simulink model "scaler_16bits_v2"  (R2021a)
settings: Solver=VariableStepAuto  StartTime=0.0  StopTime=10.0  RelTol=1e-3
libraries: xbsIndex_r4 x70
settings Model: Creator=11037  LastModifiedBy=11037

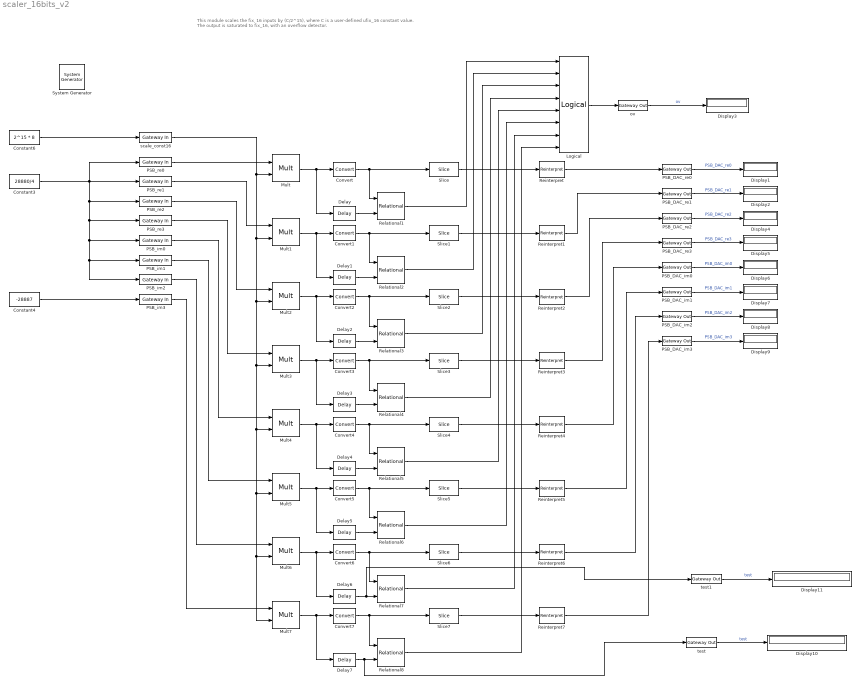
== system scaler_16bits_v2 ==
  note: This module scales the fix_16 inputs by (C/2^15),
      | where C is a user-defined ufix_16 constant value.
      | The output is saturated to fix_16, with an overflow detector.
  " System Generator" : xbsIndex_r4/ System Generator  Tag=genX  xilinxfamily=zynquplusRFSOC  part=xczu28dr  speed=-2-e  package=ffvg1517  synthesis_tool=Vivado  clock_wrapper=Clock Enables  directory=C:/scaler_16bits_v2_NL  proj_type=Vivado  Synth_file=Vivado Synthesis Defaults  Impl_file=Vivado Implementation Defaults  testbench=off  simulink_period=1  sysclk_period=10  dcm_input_clock_period=10  incr_netlist=off  trim_vbits=Everywhere in SubSystem  dbl_ovrd=According to Block Masks  core_generation=According to Block Masks  run_coregen=off  deprecated_control=off  eval_field=0  block_type=sysgen
  Constant3 : Constant  Value=28880/4  SampleTime=1
  Constant4 : Constant  Value=-28887  SampleTime=1
  Constant6 : Constant  Value=2^15 * 8  SampleTime=1
  Convert{,1..7} (8 alike) : xbsIndex_r4/Convert  gui_display_data_type=Fixed-point  arith_type="Signed  (2's comp)"  n_bits=16+15  bin_pt=0  float_type=Single  exp_bits=8  fraction_bits=24  quantization=Truncate  overflow=Saturate  en=off  latency=1  pipeline=off  dbl_ovrd=off  block_type=convert
  Delay{,1..7} (8 alike) : xbsIndex_r4/Delay  rst=off  infoeditControl=Selection of Reset will increase slice count due to use of real FFs and instead of SRLs  en=off  latency=1  reg_retiming=off  dbl_ovrd=off  block_type=delay
  Display{1..11} (11 alike) : Display
      Display1 settings: Format=decimal (Stored Integer)
      Display10 settings: Format=decimal (Stored Integer)
      Display11 settings: Format=decimal (Stored Integer)
      Display2 settings: Format=decimal (Stored Integer)
      Display3 settings: Format=binary (Stored Integer)
      Display4 settings: Format=decimal (Stored Integer)
      Display5 settings: Format=decimal (Stored Integer)
      Display6 settings: Format=decimal (Stored Integer)
      Display7 settings: Format=decimal (Stored Integer)
      Display8 settings: Format=decimal (Stored Integer)
      Display9 settings: Format=decimal (Stored Integer)
  Logical : xbsIndex_r4/Logical  logical_function=OR  inputs=8  en=off  latency=1  precision=User Defined  arith_type=Boolean  n_bits=1  bin_pt=0  align_bp=on  dbl_ovrd=off  block_type=logical
  Mult{,1..7} (8 alike) : xbsIndex_r4/Mult  precision=User Defined  arith_type="Signed  (2's comp)"  n_bits=48  bin_pt=0  quantization=Truncate  overflow=Flag as error  en=off  latency=3  use_behavioral_HDL=off  opt=Speed  use_embedded=on  optimum_pipeline=off  pipeline=on  dbl_ovrd=off  use_rpm=on  placement_style=Triangular  block_type=mult
  PSB_DAC_im{0..3} (4 alike) : xbsIndex_r4/Gateway Out  inherit_from_input=on  hdl_port=on  rows=1  columns=1  UseAsDAC=off  DACChannel='1'  interface=None  automatic_assignment=on  address_offset=hex2dec('00')  intf_name=''  intf_description=''  timing_constraint=None  locs_specified=off  LOCs={}  io_standard={}  block_type=gatewayout
  PSB_DAC_re{0..3} (4 alike) : xbsIndex_r4/Gateway Out  inherit_from_input=on  hdl_port=on  rows=1  columns=1  UseAsDAC=off  DACChannel='1'  interface=None  automatic_assignment=on  address_offset=hex2dec('00')  intf_name=''  intf_description=''  timing_constraint=None  locs_specified=off  LOCs={}  io_standard={}  block_type=gatewayout
  PSB_im{0..3} (4 alike) : xbsIndex_r4/Gateway In  gui_display_data_type=Fixed-point  arith_type="Signed  (2's comp)"  n_bits=16  bin_pt=0  preci_type=Single  exp_width=8  frac_width=24  rows=1  columns=1  quantization=Truncate  overflow=Saturate  period=1  UseAsADC=off  ADCChannel='1'  interface=None  automatic_assignment=on  address_offset=hex2dec('00')  intf_name=''  intf_description=''  default_value=0  timing_constraint=None  locs_specified=off  LOCs={}  io_standard={}  inherit_from_input=off  hdl_port=on  dbl_ovrd=off  block_type=gatewayin
  PSB_re{0..3} (4 alike) : xbsIndex_r4/Gateway In  gui_display_data_type=Fixed-point  arith_type="Signed  (2's comp)"  n_bits=16  bin_pt=0  preci_type=Single  exp_width=8  frac_width=24  rows=1  columns=1  quantization=Truncate  overflow=Saturate  period=1  UseAsADC=off  ADCChannel='1'  interface=None  automatic_assignment=on  address_offset=hex2dec('00')  intf_name=''  intf_description=''  default_value=0  timing_constraint=None  locs_specified=off  LOCs={}  io_standard={}  inherit_from_input=off  hdl_port=on  dbl_ovrd=off  block_type=gatewayin
  Reinterpret{,1..7} (8 alike) : xbsIndex_r4/Reinterpret  force_arith_type=on  arith_type="Signed  (2's comp)"  force_bin_pt=off  bin_pt=0  block_type=reinterpret
  Relational{1..8} (8 alike) : xbsIndex_r4/Relational  mode=a!=b  op_type=Bool  en=off  latency=1  dbl_ovrd=off  block_type=relational
  Slice{,1..7} (8 alike) : xbsIndex_r4/Slice  nbits=16  boolean_output=off  mode=Upper Bit Location + Width  bit1=0  base1=MSB of Input  bit0=0  base0=LSB of Input  dbl_ovrd=off  block_type=slice
  ov : xbsIndex_r4/Gateway Out  inherit_from_input=on  hdl_port=on  rows=1  columns=1  UseAsDAC=off  DACChannel='1'  interface=None  automatic_assignment=on  address_offset=hex2dec('00')  intf_name=''  intf_description=''  timing_constraint=None  locs_specified=off  LOCs={}  io_standard={}  block_type=gatewayout
  scale_const16 : xbsIndex_r4/Gateway In  gui_display_data_type=Fixed-point  arith_type=Unsigned  n_bits=32  bin_pt=0  preci_type=Single  exp_width=8  frac_width=24  rows=1  columns=1  quantization=Truncate  overflow=Wrap  period=1  UseAsADC=off  ADCChannel='1'  interface=None  automatic_assignment=on  address_offset=hex2dec('00')  intf_name=''  intf_description=''  default_value=0  timing_constraint=None  locs_specified=off  LOCs={}  io_standard={}  inherit_from_input=off  hdl_port=on  dbl_ovrd=off  block_type=gatewayin
  test : xbsIndex_r4/Gateway Out  inherit_from_input=on  hdl_port=on  rows=1  columns=1  UseAsDAC=off  DACChannel='1'  interface=None  automatic_assignment=on  address_offset=hex2dec('00')  intf_name=''  intf_description=''  timing_constraint=None  locs_specified=off  LOCs={}  io_standard={}  block_type=gatewayout
  test1 : xbsIndex_r4/Gateway Out  inherit_from_input=on  hdl_port=on  rows=1  columns=1  UseAsDAC=off  DACChannel='1'  interface=None  automatic_assignment=on  address_offset=hex2dec('00')  intf_name=''  intf_description=''  timing_constraint=None  locs_specified=off  LOCs={}  io_standard={}  block_type=gatewayout
  wires:
  Constant3/1 -> PSB_im2/1, PSB_im1/1, PSB_im0/1, PSB_re3/1, PSB_re2/1, PSB_re1/1, PSB_re0/1
  Constant4/1 -> PSB_im3/1
  PSB_re0/1 -> Mult/1
  scale_const16/1 -> Mult7/2, Mult6/2, Mult5/2, Mult4/2, Mult3/2, Mult2/2, Mult1/2, Mult/2
  Constant6/1 -> scale_const16/1
  Mult/1 -> Delay/1, Convert/1
  Convert/1 -> Relational1/1, Slice/1
  Slice/1 -> Reinterpret/1
  PSB_DAC_re0/1 -> Display1/1  "PSB_DAC_re0"
  ov/1 -> Display3/1  "ov"
  Reinterpret/1 -> PSB_DAC_re0/1
  Slice1/1 -> Reinterpret1/1
  Convert1/1 -> Relational2/1, Slice1/1
  Mult1/1 -> Delay1/1, Convert1/1
  Slice2/1 -> Reinterpret2/1
  Convert2/1 -> Relational3/1, Slice2/1
  Mult2/1 -> Delay2/1, Convert2/1
  Slice3/1 -> Reinterpret3/1
  Convert3/1 -> Relational4/1, Slice3/1
  Mult3/1 -> Delay3/1, Convert3/1
  Slice4/1 -> Reinterpret4/1
  Convert4/1 -> Relational5/1, Slice4/1
  Mult4/1 -> Delay4/1, Convert4/1
  Slice5/1 -> Reinterpret5/1
  Convert5/1 -> Relational6/1, Slice5/1
  Mult5/1 -> Delay5/1, Convert5/1
  Slice6/1 -> Reinterpret6/1
  Convert6/1 -> Relational7/1, Slice6/1
  Mult6/1 -> Delay6/1, Convert6/1
  Slice7/1 -> Reinterpret7/1
  Convert7/1 -> Relational8/1, Slice7/1
  Mult7/1 -> Delay7/1, Convert7/1
  PSB_re1/1 -> Mult1/1
  PSB_re2/1 -> Mult2/1
  PSB_re3/1 -> Mult3/1
  PSB_im0/1 -> Mult4/1
  PSB_im1/1 -> Mult5/1
  PSB_im2/1 -> Mult6/1
  PSB_im3/1 -> Mult7/1
  Reinterpret1/1 -> PSB_DAC_re1/1
  Reinterpret2/1 -> PSB_DAC_re2/1
  Reinterpret3/1 -> PSB_DAC_re3/1
  Reinterpret4/1 -> PSB_DAC_im0/1
  Reinterpret5/1 -> PSB_DAC_im1/1
  Reinterpret6/1 -> PSB_DAC_im2/1
  Reinterpret7/1 -> PSB_DAC_im3/1
  PSB_DAC_re1/1 -> Display2/1  "PSB_DAC_re1"
  PSB_DAC_re2/1 -> Display4/1  "PSB_DAC_re2"
  PSB_DAC_re3/1 -> Display5/1  "PSB_DAC_re3"
  PSB_DAC_im0/1 -> Display6/1  "PSB_DAC_im0"
  PSB_DAC_im1/1 -> Display7/1  "PSB_DAC_im1"
  PSB_DAC_im2/1 -> Display8/1  "PSB_DAC_im2"
  PSB_DAC_im3/1 -> Display9/1  "PSB_DAC_im3"
  Relational8/1 -> Logical/8
  Relational7/1 -> Logical/7
  Relational6/1 -> Logical/6
  Relational5/1 -> Logical/5
  Relational4/1 -> Logical/4
  Relational3/1 -> Logical/3
  Relational2/1 -> Logical/2
  Relational1/1 -> Logical/1
  Logical/1 -> ov/1
  Delay/1 -> Relational1/2
  Delay1/1 -> Relational2/2
  Delay2/1 -> Relational3/2
  Delay3/1 -> Relational4/2
  Delay4/1 -> Relational5/2
  Delay5/1 -> Relational6/2
  Delay6/1 -> test1/1, Relational7/2
  Delay7/1 -> test/1, Relational8/2
  test/1 -> Display10/1  "test"
  test1/1 -> Display11/1  "test"
